simulink model "RefModel_SignalIntegrity"  (R2020a)
settings: Solver=ode1  StartTime=0.0  StopTime=10.0  FixedStep=Ts_SignalIntegrity.Ts_base  RelTol=1e-3
undefined symbols (not defined in the file or in its folder): ALGO_SET, IMU1, IMU2, IMU3, mag1, mag2, SIM_SENSOR_SET
(part 2 of 2)

== stateflow chart RefModel_SignalIntegrity/SignalIntegrityCal ==
  state FaultDetect [parallel]
    settings: executionOrder=1
    state IMU1 [parallel]
      settings: executionOrder=8
      state BaseUpdate [parallel]
        du:
        updateFlag.IMU1 = hasChanged(IN_SENSOR.IMU1.accel_x) || ...
        hasChanged(IN_SENSOR.IMU1.accel_y) || ...
        hasChanged(IN_SENSOR.IMU1.accel_z);
        settings: executionOrder=1
        state Normal
          en:
          SensorStatus.IMU1 = ENUM_SensorHealthStatus.Health;
        state Degrade
          en:
          SensorStatus.IMU1 = ENUM_SensorHealthStatus.Degrade;
        (default) -> FaultDetect.IMU1.BaseUpdate.Normal
        FaultDetect.IMU1.BaseUpdate.Degrade -> FaultDetect.IMU1.BaseUpdate.Normal : [~isMeasureAbnormal]
        FaultDetect.IMU1.BaseUpdate.Normal -> FaultDetect.IMU1.BaseUpdate.Degrade : [isMeasureAbnormal]
      state WORKING [parallel]
        settings: executionOrder=2
        state NORMAL
          en:
          sensorLostTime.IMU1 = 0;
          du:
          sensorLostTime.IMU1 = sensorLostTime.IMU1 + 1;
        state LostShort
          en:
          fprintf('\t\t\t time %.2f [sec]: IMU1 is lost shortly!\n',clock_sec);
          en,du:
          SensorStatus.IMU1 = ENUM_SensorHealthStatus.LostShort;
          sensorLostTime.IMU1 = sensorLostTime.IMU1 + 1;
        state LostLong
          en:
          fprintf('\t\t\t time %.2f [sec]: IMU1 is lost!\n',clock_sec);
          en,du:
          SensorStatus.IMU1 = ENUM_SensorHealthStatus.LostLong;
          sensorLostTime.IMU1 = sensorLostTime.IMU1 + 1;
        (default) -> FaultDetect.IMU1.WORKING.NORMAL
        (junction 288) -> FaultDetect.IMU1.WORKING.NORMAL : [updateFlag.IMU1]
            | {sensorLostTime.IMU1 = 0;}
        FaultDetect.IMU1.WORKING.NORMAL -> (junction 289) [order 1]
        FaultDetect.IMU1.WORKING.NORMAL -> FaultDetect.IMU1.WORKING.LostShort [order 2] : [sensorLostTime.IMU1 > SENSOR_INTEGRITY_PARAM.IMU.threshold_lostTime]
        (junction 289) -> (junction 288)
        (junction 290) -> (junction 288) : [updateFlag.IMU1]
            | {fprintf('\t\t\t time %.2f [sec]: IMU1 is normal!\n',clock_sec);
            | }
        FaultDetect.IMU1.WORKING.LostShort -> (junction 290) [order 1]
        FaultDetect.IMU1.WORKING.LostLong -> (junction 290)
        FaultDetect.IMU1.WORKING.LostShort -> FaultDetect.IMU1.WORKING.LostLong [order 2] : [sensorLostTime.IMU1 > 2*SENSOR_INTEGRITY_PARAM.IMU.threshold_lostTime]
    state IMU2 [parallel]
      settings: executionOrder=9
      state WORKING [parallel]
        settings: executionOrder=2
        state NORMAL
          en:
          sensorLostTime.IMU2 = 0;
          du:
          sensorLostTime.IMU2 = sensorLostTime.IMU2 + 1;
        state LostShort
          en:
          en,du:
          SensorStatus.IMU2 = ENUM_SensorHealthStatus.LostShort;
          sensorLostTime.IMU2 = sensorLostTime.IMU2 + 1;
        state LostLong
          en:
          en,du:
          SensorStatus.IMU2 = ENUM_SensorHealthStatus.LostLong;
          sensorLostTime.IMU2 = sensorLostTime.IMU2 + 1;
        (default) -> FaultDetect.IMU2.WORKING.NORMAL
        (junction 308) -> FaultDetect.IMU2.WORKING.NORMAL : [updateFlag.IMU2]
            | {sensorLostTime.IMU2 = 0;}
        FaultDetect.IMU2.WORKING.NORMAL -> (junction 309) [order 1]
        FaultDetect.IMU2.WORKING.NORMAL -> FaultDetect.IMU2.WORKING.LostShort [order 2] : [sensorLostTime.IMU2 > SENSOR_INTEGRITY_PARAM.IMU.threshold_lostTime]
        (junction 309) -> (junction 308)
        (junction 310) -> (junction 308)
        FaultDetect.IMU2.WORKING.LostShort -> (junction 310) [order 1]
        FaultDetect.IMU2.WORKING.LostLong -> (junction 310)
        FaultDetect.IMU2.WORKING.LostShort -> FaultDetect.IMU2.WORKING.LostLong [order 2] : [sensorLostTime.IMU2 > 2*SENSOR_INTEGRITY_PARAM.IMU.threshold_lostTime]
      state BaseUpdate [parallel]
        du:
        updateFlag.IMU2 = hasChanged(IN_SENSOR.IMU2.accel_x) || ...
        hasChanged(IN_SENSOR.IMU2.accel_y) || ...
        hasChanged(IN_SENSOR.IMU2.accel_z);
        if isMeasureAbnormal
        SensorStatus.IMU2 = ENUM_SensorHealthStatus.Degrade;
        else
        SensorStatus.IMU2 = ENUM_SensorHealthStatus.Health;
        end
        settings: executionOrder=1
    state IMU3 [parallel]
      settings: executionOrder=10
      state WORKING [parallel]
        settings: executionOrder=2
        state NORMAL
          en:
          sensorLostTime.IMU3 = 0;
          du:
          sensorLostTime.IMU3 = sensorLostTime.IMU3 + 1;
        state LostShort
          en:
          en,du:
          SensorStatus.IMU3 = ENUM_SensorHealthStatus.LostShort;
          sensorLostTime.IMU3 = sensorLostTime.IMU3 + 1;
        state LostLong
          en:
          en,du:
          SensorStatus.IMU3 = ENUM_SensorHealthStatus.LostLong;
          sensorLostTime.IMU3 = sensorLostTime.IMU3 + 1;
        (default) -> FaultDetect.IMU3.WORKING.NORMAL
        (junction 328) -> FaultDetect.IMU3.WORKING.NORMAL : [updateFlag.IMU3]
            | {sensorLostTime.IMU3 = 0;}
        FaultDetect.IMU3.WORKING.NORMAL -> (junction 329) [order 1]
        FaultDetect.IMU3.WORKING.NORMAL -> FaultDetect.IMU3.WORKING.LostShort [order 2] : [sensorLostTime.IMU3 > SENSOR_INTEGRITY_PARAM.IMU.threshold_lostTime]
        (junction 329) -> (junction 328)
        (junction 330) -> (junction 328)
        FaultDetect.IMU3.WORKING.LostShort -> (junction 330) [order 1]
        FaultDetect.IMU3.WORKING.LostLong -> (junction 330)
        FaultDetect.IMU3.WORKING.LostShort -> FaultDetect.IMU3.WORKING.LostLong [order 2] : [sensorLostTime.IMU3 > 2*SENSOR_INTEGRITY_PARAM.IMU.threshold_lostTime]
      state BaseUpdate [parallel]
        du:
        updateFlag.IMU3 = hasChanged(IN_SENSOR.IMU3.accel_x) || ...
        hasChanged(IN_SENSOR.IMU3.accel_y) || ...
        hasChanged(IN_SENSOR.IMU3.accel_z);
        if isMeasureAbnormal
        SensorStatus.IMU3 = ENUM_SensorHealthStatus.Degrade;
        else
        SensorStatus.IMU3 = ENUM_SensorHealthStatus.Health;
        end
        settings: executionOrder=1
    state Mag1 [parallel]
      settings: executionOrder=1
      state BaseUpdate [parallel]
        du:
        updateFlag.mag1 = hasChanged(IN_SENSOR.mag1.mag_x) || ...
        hasChanged(IN_SENSOR.mag1.mag_y) || ...
        hasChanged(IN_SENSOR.mag1.mag_z);
        settings: executionOrder=1
        state Normal
          en:
          SensorStatus.mag1 = ENUM_SensorHealthStatus.Health;
        state Degrade
          en:
          SensorStatus.mag1 = ENUM_SensorHealthStatus.Degrade;
        (default) -> FaultDetect.Mag1.BaseUpdate.Normal
        FaultDetect.Mag1.BaseUpdate.Degrade -> FaultDetect.Mag1.BaseUpdate.Normal : [~isMeasureAbnormal]
        FaultDetect.Mag1.BaseUpdate.Normal -> FaultDetect.Mag1.BaseUpdate.Degrade : [isMeasureAbnormal]
      state WORKING [parallel]
        settings: executionOrder=2
        state NORMAL
          en:
          sensorLostTime.mag1 = 0;
          SensorStatus.mag1 = ENUM_SensorHealthStatus.Health;
          du:
          sensorLostTime.mag1 = sensorLostTime.mag1 + 1;
        state LostShort
          en:
          fprintf('\t\t\t time %.2f [sec]: Mag1 is lost shortly!\n',clock_sec);
          en,du:
          SensorStatus.mag1 = ENUM_SensorHealthStatus.LostShort;
          sensorLostTime.mag1 = sensorLostTime.mag1 + 1;
        state LostLong
          en:
          fprintf('\t\t\t time %.2f [sec]: Mag1 is lost!\n',clock_sec);
          en,du:
          SensorStatus.mag1 = ENUM_SensorHealthStatus.LostLong;
          sensorLostTime.mag1 = sensorLostTime.mag1 + 1;
        (default) -> FaultDetect.Mag1.WORKING.NORMAL
        (junction 65) -> FaultDetect.Mag1.WORKING.NORMAL : [updateFlag.mag1]
            | {sensorLostTime.mag1 = 0;}
        FaultDetect.Mag1.WORKING.NORMAL -> (junction 66) [order 1]
        FaultDetect.Mag1.WORKING.NORMAL -> FaultDetect.Mag1.WORKING.LostShort [order 2] : [sensorLostTime.mag1 > SENSOR_INTEGRITY_PARAM.Mag.threshold_lostTime]
        (junction 66) -> (junction 65)
        (junction 156) -> (junction 65) : [updateFlag.mag1]
            | {
            | fprintf('\t\t\t time %.2f [sec]: Mag1 is normal!\n',clock_sec);
            | }
        FaultDetect.Mag1.WORKING.LostShort -> (junction 156) [order 1]
        FaultDetect.Mag1.WORKING.LostLong -> (junction 156)
        FaultDetect.Mag1.WORKING.LostShort -> FaultDetect.Mag1.WORKING.LostLong [order 2] : [sensorLostTime.mag1 > 2*SENSOR_INTEGRITY_PARAM.Mag.threshold_lostTime]
    state Mag2 [parallel]
      settings: executionOrder=2
      state BaseUpdate [parallel]
        du:
        updateFlag.mag2 = hasChanged(IN_SENSOR.mag2.mag_x) || ...
        hasChanged(IN_SENSOR.mag2.mag_y) || ...
        hasChanged(IN_SENSOR.mag2.mag_z);
        settings: executionOrder=1
        state Normal
          en:
          SensorStatus.mag2 = ENUM_SensorHealthStatus.Health;
        state Degrade
          en:
          SensorStatus.mag2 = ENUM_SensorHealthStatus.Degrade;
        (default) -> FaultDetect.Mag2.BaseUpdate.Normal
        FaultDetect.Mag2.BaseUpdate.Degrade -> FaultDetect.Mag2.BaseUpdate.Normal : [~isMeasureAbnormal]
        FaultDetect.Mag2.BaseUpdate.Normal -> FaultDetect.Mag2.BaseUpdate.Degrade : [isMeasureAbnormal]
      state WORKING [parallel]
        settings: executionOrder=2
        state NORMAL
          en:
          sensorLostTime.mag2 = 0;
          SensorStatus.mag2 = ENUM_SensorHealthStatus.Health;
          du:
          sensorLostTime.mag2 = sensorLostTime.mag2 + 1;
        state LostShort
          en:
          fprintf('\t\t\t time %.2f [sec]: Mag2 is lost shortly!\n',clock_sec);
          en,du:
          SensorStatus.mag2 = ENUM_SensorHealthStatus.LostShort;
          sensorLostTime.mag2 = sensorLostTime.mag2 + 1;
        state LostLong
          en:
          fprintf('\t\t\t time %.2f [sec]: Mag2 is lost!\n',clock_sec);
          en,du:
          SensorStatus.mag2 = ENUM_SensorHealthStatus.LostLong;
          sensorLostTime.mag2 = sensorLostTime.mag2 + 1;
        (default) -> FaultDetect.Mag2.WORKING.NORMAL
        (junction 168) -> FaultDetect.Mag2.WORKING.NORMAL : [updateFlag.mag2]
            | {sensorLostTime.mag2 = 0;}
        FaultDetect.Mag2.WORKING.NORMAL -> (junction 169) [order 1]
        FaultDetect.Mag2.WORKING.NORMAL -> FaultDetect.Mag2.WORKING.LostShort [order 2] : [sensorLostTime.mag2 > SENSOR_INTEGRITY_PARAM.Mag.threshold_lostTime]
        (junction 169) -> (junction 168)
        (junction 170) -> (junction 168) : [updateFlag.mag2]
            | {
            | fprintf('\t\t\t time %.2f [sec]: Mag2 is normal!\n',clock_sec);
            | }
        FaultDetect.Mag2.WORKING.LostShort -> (junction 170) [order 1]
        FaultDetect.Mag2.WORKING.LostLong -> (junction 170)
        FaultDetect.Mag2.WORKING.LostShort -> FaultDetect.Mag2.WORKING.LostLong [order 2] : [sensorLostTime.mag2 > 2*SENSOR_INTEGRITY_PARAM.Mag.threshold_lostTime]
    state Ublox1 [parallel]
      settings: executionOrder=3
      state WORKING [parallel]
        settings: executionOrder=2
        state NORMAL
          en:
          sensorLostTime.ublox1 = 0;
          du:
          sensorLostTime.ublox1 = sensorLostTime.ublox1 + 1;
        state LostShort
          en:
          fprintf('\t\t\t time %.2f [sec]: Ublox1 is lost shortly!\n',clock_sec);
          en,du:
          SensorStatus.ublox1 = ENUM_SensorHealthStatus.LostShort;
          sensorLostTime.ublox1 = sensorLostTime.ublox1 + 1;
        state LostLong
          en:
          fprintf('\t\t\t time %.2f [sec]: Ublox1 is lost!\n',clock_sec);
          en,du:
          SensorStatus.ublox1 = ENUM_SensorHealthStatus.LostLong;
          sensorLostTime.ublox1 = sensorLostTime.ublox1 + 1;
        (default) -> FaultDetect.Ublox1.WORKING.NORMAL
        (junction 188) -> FaultDetect.Ublox1.WORKING.NORMAL : [updateFlag.ublox1]
            | {sensorLostTime.ublox1 = 0;}
        FaultDetect.Ublox1.WORKING.NORMAL -> (junction 189) [order 1]
        FaultDetect.Ublox1.WORKING.NORMAL -> FaultDetect.Ublox1.WORKING.LostShort [order 2] : [sensorLostTime.ublox1 > SENSOR_INTEGRITY_PARAM.GPS.threshold_lostTime]
        (junction 189) -> (junction 188)
        (junction 190) -> (junction 188) : [updateFlag.ublox1]
            | {fprintf('\t\t\t time %.2f [sec]: Ublox1 is normal!\n',clock_sec);
            | }
        FaultDetect.Ublox1.WORKING.LostShort -> (junction 190) [order 1]
        FaultDetect.Ublox1.WORKING.LostLong -> (junction 190)
        FaultDetect.Ublox1.WORKING.LostShort -> FaultDetect.Ublox1.WORKING.LostLong [order 2] : [sensorLostTime.ublox1 > 2*SENSOR_INTEGRITY_PARAM.GPS.threshold_lostTime]
      state BaseUpdate [parallel]
        du:
        updateFlag.ublox1 = hasChanged(IN_SENSOR.ublox1.velN) || ...
        hasChanged(IN_SENSOR.ublox1.velE) || ...
        hasChanged(IN_SENSOR.ublox1.velD);
        if isMeasureAbnormal
        SensorStatus.ublox1 = ENUM_SensorHealthStatus.Degrade;
        else
        SensorStatus.ublox1 = ENUM_SensorHealthStatus.Health;
        end
        settings: executionOrder=1
    state BoardCard [parallel]
      settings: executionOrder=4
      state WORKING [parallel]
        settings: executionOrder=2
        state NORMAL
          en:
          sensorLostTime.um482 = 0;
          du:
          sensorLostTime.um482 = sensorLostTime.um482 + 1;
        state LostShort
          en,du:
          SensorStatus.um482 = ENUM_SensorHealthStatus.LostShort;
          sensorLostTime.um482 = sensorLostTime.um482 + 1;
        state LostLong
          en:
          fprintf('\t\t\t time %.2f [sec]: um482 is lost!\n',clock_sec);
          en,du:
          SensorStatus.um482 = ENUM_SensorHealthStatus.LostLong;
          sensorLostTime.um482 = sensorLostTime.um482 + 1;
        (default) -> FaultDetect.BoardCard.WORKING.NORMAL
        (junction 208) -> FaultDetect.BoardCard.WORKING.NORMAL : [updateFlag.um482]
            | {sensorLostTime.um482 = 0;}
        FaultDetect.BoardCard.WORKING.NORMAL -> (junction 209) [order 1]
        FaultDetect.BoardCard.WORKING.NORMAL -> FaultDetect.BoardCard.WORKING.LostShort [order 2] : [sensorLostTime.um482 > SENSOR_INTEGRITY_PARAM.um482.threshold_lostTime]
        (junction 209) -> (junction 208)
        (junction 210) -> (junction 208) : [updateFlag.um482]
            | {fprintf('\t\t\t time %.2f [sec]: um482 is normal!\n',clock_sec);
            | }
        FaultDetect.BoardCard.WORKING.LostShort -> (junction 210) [order 1]
        FaultDetect.BoardCard.WORKING.LostLong -> (junction 210)
        FaultDetect.BoardCard.WORKING.LostShort -> FaultDetect.BoardCard.WORKING.LostLong [order 2] : [sensorLostTime.um482 > 2*SENSOR_INTEGRITY_PARAM.um482.threshold_lostTime]
      state BaseUpdate [parallel]
        en,du:
        updateBESTPOS;
        updateFlag.um482 = hasChanged(IN_SENSOR.um482.velN) || ...
        hasChanged(IN_SENSOR.um482.velE) || ...
        hasChanged(IN_SENSOR.um482.velD);
        if isMeasureAbnormal
        SensorStatus.um482 = ENUM_SensorHealthStatus.Degrade;
        else
        SensorStatus.um482 = ENUM_SensorHealthStatus.Health;
        end
        settings: executionOrder=1
    state Baro1 [parallel]
      settings: executionOrder=5
      state WORKING [parallel]
        settings: executionOrder=2
        state NORMAL
          en:
          sensorLostTime.baro1 = 0;
          du:
          sensorLostTime.baro1 = sensorLostTime.baro1 + 1;
        state LostShort
          en:
          fprintf('\t\t\t time %.2f [sec]: Baro1 is lost shortly!\n',clock_sec);
          en,du:
          SensorStatus.baro1 = ENUM_SensorHealthStatus.LostShort;
          sensorLostTime.baro1 = sensorLostTime.baro1 + 1;
        state LostLong
          en:
          fprintf('\t\t\t time %.2f [sec]: Baro1 is lost!\n',clock_sec);
          en,du:
          SensorStatus.baro1 = ENUM_SensorHealthStatus.LostLong;
          sensorLostTime.baro1 = sensorLostTime.baro1 + 1;
        (default) -> FaultDetect.Baro1.WORKING.NORMAL
        (junction 228) -> FaultDetect.Baro1.WORKING.NORMAL : [updateFlag.baro1]
            | {sensorLostTime.baro1 = 0;}
        FaultDetect.Baro1.WORKING.NORMAL -> (junction 229) [order 1]
        FaultDetect.Baro1.WORKING.NORMAL -> FaultDetect.Baro1.WORKING.LostShort [order 2] : [sensorLostTime.baro1 > SENSOR_INTEGRITY_PARAM.Baro.threshold_lostTime]
        (junction 229) -> (junction 228)
        (junction 230) -> (junction 228) : [updateFlag.baro1]
            | {fprintf('\t\t\t time %.2f [sec]: Baro1 is normal!\n',clock_sec);
            | }
        FaultDetect.Baro1.WORKING.LostShort -> (junction 230) [order 1]
        FaultDetect.Baro1.WORKING.LostLong -> (junction 230)
        FaultDetect.Baro1.WORKING.LostShort -> FaultDetect.Baro1.WORKING.LostLong [order 2] : [sensorLostTime.baro1 > 2*SENSOR_INTEGRITY_PARAM.Baro.threshold_lostTime]
      state BaseUpdate [parallel]
        du:
        updateFlag.baro1 = hasChanged(IN_SENSOR.baro1.alt_baro);
        if isMeasureAbnormal
        SensorStatus.baro1 = ENUM_SensorHealthStatus.Degrade;
        else
        SensorStatus.baro1 = ENUM_SensorHealthStatus.Health;
        end
        settings: executionOrder=1
    state Radar1 [parallel]
      settings: executionOrder=6
      state WORKING [parallel]
        settings: executionOrder=2
        state NORMAL
          en:
          sensorLostTime.radar1 = 0;
          du:
          sensorLostTime.radar1 = sensorLostTime.radar1 + 1;
        state LostShort
          en:
          fprintf('\t\t\t time %.2f [sec]: Radar1 is lost shortly!\n',clock_sec);
          en,du:
          SensorStatus.radar1 = ENUM_SensorHealthStatus.LostShort;
          sensorLostTime.radar1 = sensorLostTime.radar1 + 1;
        state LostLong
          en:
          fprintf('\t\t\t time %.2f [sec]: Radar1 is lost!\n',clock_sec);
          en,du:
          SensorStatus.radar1 = ENUM_SensorHealthStatus.LostLong;
          sensorLostTime.radar1 = sensorLostTime.radar1 + 1;
        (default) -> FaultDetect.Radar1.WORKING.NORMAL
        (junction 248) -> FaultDetect.Radar1.WORKING.NORMAL : [updateFlag.radar1]
            | {sensorLostTime.radar1 = 0;}
        FaultDetect.Radar1.WORKING.NORMAL -> (junction 249) [order 1]
        FaultDetect.Radar1.WORKING.NORMAL -> FaultDetect.Radar1.WORKING.LostShort [order 2] : [sensorLostTime.radar1 > SENSOR_INTEGRITY_PARAM.Radar.threshold_lostTime]
        (junction 249) -> (junction 248)
        (junction 250) -> (junction 248) : [updateFlag.radar1]
            | {fprintf('\t\t\t time %.2f [sec]: Radar1 is normal!\n',clock_sec);
            | }
        FaultDetect.Radar1.WORKING.LostShort -> (junction 250) [order 1]
        FaultDetect.Radar1.WORKING.LostLong -> (junction 250)
        FaultDetect.Radar1.WORKING.LostShort -> FaultDetect.Radar1.WORKING.LostLong [order 2] : [sensorLostTime.radar1 > 2*SENSOR_INTEGRITY_PARAM.Radar.threshold_lostTime]
      state BaseUpdate [parallel]
        du:
        updateFlag.radar1 = hasChanged(IN_SENSOR.radar1.Range);
        if isMeasureAbnormal
        SensorStatus.radar1 = ENUM_SensorHealthStatus.Degrade;
        else
        SensorStatus.radar1 = ENUM_SensorHealthStatus.Health;
        end
        settings: executionOrder=1
    state Airspeed1 [parallel]
      settings: executionOrder=7
      state WORKING [parallel]
        settings: executionOrder=2
        state NORMAL
          en:
          sensorLostTime.airspeed1 = 0;
          du:
          sensorLostTime.airspeed1 = sensorLostTime.airspeed1 + 1;
        state LostShort
          en:
          fprintf('\t\t\t time %.2f [sec]: Airspeed is lost shortly!\n',clock_sec);
          en,du:
          SensorStatus.airspeed1 = ENUM_SensorHealthStatus.LostShort;
          sensorLostTime.airspeed1 = sensorLostTime.airspeed1 + 1;
        state LostLong
          en:
          fprintf('\t\t\t time %.2f [sec]: Airspeed1 is lost!\n',clock_sec);
          en,du:
          SensorStatus.airspeed1 = ENUM_SensorHealthStatus.LostLong;
          sensorLostTime.airspeed1 = sensorLostTime.airspeed1 + 1;
        (default) -> FaultDetect.Airspeed1.WORKING.NORMAL
        (junction 268) -> FaultDetect.Airspeed1.WORKING.NORMAL : [updateFlag.airspeed1]
            | {sensorLostTime.airspeed1 = 0;}
        FaultDetect.Airspeed1.WORKING.NORMAL -> (junction 269) [order 1]
        FaultDetect.Airspeed1.WORKING.NORMAL -> FaultDetect.Airspeed1.WORKING.LostShort [order 2] : [sensorLostTime.airspeed1 > SENSOR_INTEGRITY_PARAM.Airspeed.threshold_lostTime]
        (junction 269) -> (junction 268)
        (junction 270) -> (junction 268) : [updateFlag.airspeed1]
            | {fprintf('\t\t\t time %.2f [sec]: Airspeed1 is normal!\n',clock_sec);
            | }
        FaultDetect.Airspeed1.WORKING.LostShort -> (junction 270) [order 1]
        FaultDetect.Airspeed1.WORKING.LostLong -> (junction 270)
        FaultDetect.Airspeed1.WORKING.LostShort -> FaultDetect.Airspeed1.WORKING.LostLong [order 2] : [sensorLostTime.airspeed1 > 2*SENSOR_INTEGRITY_PARAM.Airspeed.threshold_lostTime]
      state BaseUpdate [parallel]
        du:
        updateFlag.airspeed1 = hasChanged(IN_SENSOR.airspeed1.airspeed);
        if isMeasureAbnormal
        SensorStatus.airspeed1 = ENUM_SensorHealthStatus.Degrade;
        else
        SensorStatus.airspeed1 = ENUM_SensorHealthStatus.Health;
        end
        settings: executionOrder=1
  state OUTPUT [parallel]
    du:
    % 信号更新
    SensorIntegrityInfo.SensorUpdateFlag = updateFlag;
    % 传感器选择
    SensorIntegrityInfo.SensorSelect = selectSensorByHealth;
    % 信号丢失信息
    SensorIntegrityInfo.sensorLostTime = sensorLostTime;
    % 信号丢失信息
    SensorIntegrityInfo.SensorStatus = SensorStatus;
    % 信号丢失信息
    SensorIntegrityInfo.SystemHealthStatus = calSystemHealthStatus;
    % ECAS
    updateECASInfo;
    settings: executionOrder=2
  data: flag function_output; flag function_output; flag function_output; flag function_output; flag function_output; flag function_output; flag function_output; flag function_output; flag function_output; flag function_output; SystemHealthStatus_out function_output; out function_output; IN_SENSOR input Bus: BUS_SENSOR size=1; SensorSelect input Bus: BUS_NAVI_SensorSignalIntegrity_SensorSelect size=1; SensorIntegrityInfo output Bus: BUS_NAVI_SensorSignalIntegrity size=1; updateFlag local Bus: BUS_NAVI_SensorSignalIntegrity_SensorUpdateFlag size=1; sensorLostTime local Bus: BUS_NAVI_SensorSignalIntegrity_sensorLostTime size=1; SENSOR_INTEGRITY_PARAM parameter Bus: BUS_SENSOR_INTEGRITY_PARAM size=1; SensorStatus local Bus: BUS_NAVI_SensorSignalIntegrity_Status size=1; clock_sec input; Ts input; ECASInfo output Bus: BUS_ECAS_SingalIntegrity size=1
  function flag = isMeasureAbnormal:
    | function flag = isMeasureAbnormal
    | flag = false;
  function flag = isMeasureAbnormal:
    | function flag = isMeasureAbnormal
    | flag = false;
  function flag = isMeasureAbnormal:
    | function flag = isMeasureAbnormal
    | flag = false;
  function flag = isMeasureAbnormal:
    | function flag = isMeasureAbnormal
    | persistent normMag_pre maxMag_pre minMag_pre errIdx
    | normMag = double(norm([IN_SENSOR.mag1.mag_x,IN_SENSOR.mag1.mag_y,IN_SENSOR.mag1.mag_z]));
    | if isempty(normMag_pre)
    |     normMag_pre = normMag;
    |     maxMag_pre = normMag;
    |     minMag_pre = normMag;
    |     errIdx = 0;
    | end
    | if normMag < minMag_pre % 更新最小值
    |     minMag_pre = normMag;
    | end
    | if normMag > maxMag_pre % 更新最大值
    |     maxMag_pre = normMag;
    | end
    | flag = false;
    | if normMag < SENSOR_INTEGRITY_PARAM.Mag.threshold_minNormMag_uT || ...
    |         normMag > SENSOR_INTEGRITY_PARAM.Mag.threshold_maxNormMag_uT || ...
    |            normMag - normMag_pre > SENSOR_INTEGRITY_PARAM.Mag.threshold_gapBetweenMaxMin_uT
    |     errIdx = errIdx + Ts;
    |     if errIdx > 1
    |         flag = true; 
    |     end
    | end
    | normMag_pre = normMag;
  function flag = isMeasureAbnormal:
    | function flag = isMeasureAbnormal
    | persistent normMag_pre maxMag_pre minMag_pre errIdx
    | normMag = double(norm([IN_SENSOR.mag2.mag_x,IN_SENSOR.mag2.mag_y,IN_SENSOR.mag2.mag_z]));
    | if isempty(normMag_pre)
    |     normMag_pre = normMag;
    |     maxMag_pre = normMag;
    |     minMag_pre = normMag;
    |     errIdx = 0;
    | end
    | if normMag < minMag_pre % 更新最小值
    |     minMag_pre = normMag;
    | end
    | if normMag > maxMag_pre % 更新最大值
    |     maxMag_pre = normMag;
    | end
    | flag = false;
    | if normMag < SENSOR_INTEGRITY_PARAM.Mag.threshold_minNormMag_uT || ...
    |         normMag > SENSOR_INTEGRITY_PARAM.Mag.threshold_maxNormMag_uT || ...
    |            normMag - normMag_pre > SENSOR_INTEGRITY_PARAM.Mag.threshold_gapBetweenMaxMin_uT
    |     errIdx = errIdx + Ts;
    |     if errIdx > 1
    |         flag = true; 
    |     end
    | end
    | normMag_pre = normMag;
  function flag = isMeasureAbnormal:
    | function flag = isMeasureAbnormal
    | persistent lat_pre lon_pre speed_pre errIdx
    | tempGPS = IN_SENSOR.ublox1;
    | curLat = double(tempGPS.Lat);
    | curLon = double(tempGPS.Lon);
    | curSpeed = double(norm([tempGPS.velN,tempGPS.velE,tempGPS.velD]));
    | if isempty(lat_pre)
    |     lat_pre = curLat;
    |     lon_pre = curLon;
    |     speed_pre = curSpeed;
    |     errIdx = 0;
    | end
    | 
    | flag = false;
    | if tempGPS.numSv < SENSOR_INTEGRITY_PARAM.GPS.threshold_numSv || ...
    |         tempGPS.pDop > SENSOR_INTEGRITY_PARAM.GPS.threshold_pDop || ...
    |         abs(lat_pre-curLat) > 5e-4 || ...
    |         abs(lon_pre-curLon) > 5e-4 || ...
    |         abs(speed_pre-curSpeed) > 10
    |     errIdx = errIdx + Ts;
    |     if errIdx > 5
    |         flag = true; 
    |     end
    | else
    |     errIdx = 0;
    | end
    | 
    | lat_pre = curLat;
    | lon_pre = curLon;
    | speed_pre = curSpeed;
  function flag = isMeasureAbnormal:
    | function flag = isMeasureAbnormal
    | persistent lat_pre lon_pre speed_pre errIdx
    | tempGPS = IN_SENSOR.um482;
    | curLat = double(tempGPS.Lat);
    | curLon = double(tempGPS.Lon);
    | curSpeed = double(norm([tempGPS.velN,tempGPS.velE,tempGPS.velD]));
    | if isempty(lat_pre)
    |     lat_pre = curLat;
    |     lon_pre = curLon;
    |     speed_pre = curSpeed;
    |     errIdx = 0;
    | end
    | 
    | flag = false;
    | if tempGPS.numSv < SENSOR_INTEGRITY_PARAM.um482.threshold_numSv || ...
    |         tempGPS.pDop > SENSOR_INTEGRITY_PARAM.um482.threshold_pDop || ...
    |         abs(lat_pre-curLat) > 5e-4 || ...
    |         abs(lon_pre-curLon) > 5e-4 || ...
    |         abs(speed_pre-curSpeed) > 20
    |     errIdx = errIdx + Ts;
    |     if errIdx > 5
    |         flag = true; 
    |     end
    | else
    |     errIdx = 0;
    | end
    | 
    | lat_pre = curLat;
    | lon_pre = curLon;
    | speed_pre = curSpeed;
  function updateBESTPOS:
    | function updateBESTPOS
  function flag = isMeasureAbnormal:
    | function flag = isMeasureAbnormal
    | persistent preHeight
    | if isempty(preHeight)
    |     preHeight = 0; 
    | end
    | flag = false;
    | if abs(preHeight-IN_SENSOR.baro1.alt_baro) > 10
    |     flag = true; 
    | end
    | preHeight = double(IN_SENSOR.baro1.alt_baro);
  function flag = isMeasureAbnormal:
    | function flag = isMeasureAbnormal
    | persistent preVal
    | if isempty(preVal)
    |     preVal = IN_SENSOR.radar1.Range;
    | end
    | flag = false;
    | if abs(preVal-IN_SENSOR.radar1.Range)>10
    |     flag = true;
    | end
    | preVal = IN_SENSOR.radar1.Range;
  function flag = isMeasureAbnormal:
    | function flag = isMeasureAbnormal
    | flag = false;
  function SystemHealthStatus_out = calSystemHealthStatus:
    | function SystemHealthStatus_out = calSystemHealthStatus
    | SystemHealthStatus_out = ENUM_SystemHealthStatus.SystemHealth;
    | if SensorIntegrityInfo.SensorStatus.IMU1 == ENUM_SensorHealthStatus.Health && ...
    |         (SensorIntegrityInfo.SensorStatus.ublox1 == ENUM_SensorHealthStatus.Health)
    |     %         SensorIntegrityInfo.SensorStatus.mag2 == ENUM_SensorHealthStatus.Health && ...
    |     %         SensorIntegrityInfo.SensorStatus.baro1 == ENUM_SensorHealthStatus.Health
    |     SystemHealthStatus_out = ENUM_SystemHealthStatus.SystemHealth;
    | elseif SensorIntegrityInfo.SensorStatus.IMU1 == ENUM_SensorHealthStatus.Health && ...
    |         (SensorIntegrityInfo.SensorStatus.ublox1 ~= ENUM_SensorHealthStatus.Health && ...
    |          SensorIntegrityInfo.SensorStatus.um482 == ENUM_SensorHealthStatus.Health)
    |     SystemHealthStatus_out = ENUM_SystemHealthStatus.DontTakeOff;
    | else
    |     SystemHealthStatus_out = ENUM_SystemHealthStatus.CanNotFly;
    | end
  function out = selectSensorByHealth:
    | function out = selectSensorByHealth
    | out = SensorSelect;
    | %% 磁力计信号优选
    | if SensorStatus.mag2 == ENUM_SensorHealthStatus.Health % 磁力计2健康
    |     out.Mag = single(2);
    | elseif  SensorStatus.mag1 == ENUM_SensorHealthStatus.Health
    |     out.Mag = single(1);
    | else
    |     out.Mag = single(-1);
    | end
  function updateECASInfo:
    | function updateECASInfo
    | % 磁力计
    | if SensorStatus.mag1 == ENUM_SensorHealthStatus.Degrade || ...
    |         SensorStatus.mag2 == ENUM_SensorHealthStatus.Degrade
    |     ECASInfo.anyDegrade_mag = int8(1);
    | end
    | % 
    | mag1Val = [IN_SENSOR.mag1.mag_x,IN_SENSOR.mag1.mag_y,IN_SENSOR.mag1.mag_z];
    | mag2Val = [IN_SENSOR.mag2.mag_x,IN_SENSOR.mag2.mag_y,IN_SENSOR.mag2.mag_z];
    | if norm(mag1Val-mag2Val) > 0.15*min(norm(mag1Val),norm(mag2Val))
    |     ECASInfo.precisionMismatch_mag = int8(1);
    | end
  function getSensorSignalBySelect:
    | function getSensorSignalBySelect
    | % IMU更新
    | if SensorIntegrityInfo.SensorSelect.IMU == 1
    |     imuUpdateFlag = SensorIntegrityInfo.SensorUpdateFlag.IMU1;
    |     accel = IMU1_accel;
    |     gyro = IMU1_gyro;
    | elseif SensorIntegrityInfo.SensorSelect.IMU == 2
    |     imuUpdateFlag = SensorIntegrityInfo.SensorUpdateFlag.IMU2;
    |     accel = IMU2_accel;
    |     gyro = IMU2_gyro;
    | elseif SensorIntegrityInfo.SensorSelect.IMU == 3
    |     imuUpdateFlag = SensorIntegrityInfo.SensorUpdateFlag.IMU3;
    |     accel = IMU3_accel;
    |     gyro = IMU3_gyro;
    | elseif SensorIntegrityInfo.SensorSelect.IMU == 0
    |     imuUpdateFlag = SensorIntegrityInfo.SensorUpdateFlag.IMU1 & SensorIntegrityInfo.SensorUpdateFlag.IMU2 & SensorIntegrityInfo.SensorUpdateFlag.IMU3;
    |     accel = (IMU1_accel+IMU2_accel+IMU3_accel)/3;
    |     gyro = (IMU1_gyro+IMU2_gyro+IMU3_gyro)/3;
    | else
    |     imuUpdateFlag = true;
    |     accelTemp = single([0,0,0]);
    |     gyroTemp = single([0,0,0]);
    |     error('IMU config error')
    | end
    | % Mag更新
    | if SensorIntegrityInfo.SensorSelect.Mag == 1
    |     magUpdateFlag = SensorIntegrityInfo.SensorUpdateFlag.mag1;
    |     mag = mag1;
    | elseif SensorIntegrityInfo.SensorSelect.Mag == 2
    |     magUpdateFlag = SensorIntegrityInfo.SensorUpdateFlag.mag2;
    |     mag = mag2;
    | elseif SensorIntegrityInfo.SensorSelect.Mag == 0
    |     magUpdateFlag = SensorIntegrityInfo.SensorUpdateFlag.mag1 & SensorIntegrityInfo.SensorUpdateFlag.mag2;
    |     mag = (mag1+mag2)/2;
    | else % 随便预置一个地磁矢量
    |     magUpdateFlag = true;
    |     mag = [1,0,0];
    | end
    | % GPS更新
    | lla = ublox1_lla;
    | gpsvel = ublox1_gpsvel;
    | gpsUpdateFlag = SensorIntegrityInfo.SensorUpdateFlag.ublox1;
    | % 气压高度计更新
    | alt = baro1_alt;
    | baroUpdateFlag = SensorIntegrityInfo.SensorUpdateFlag.baro1;
    | % 雷达高度计更新
    | range = radar1_range;
    | radarUpdateFlag = SensorIntegrityInfo.SensorUpdateFlag.radar1;

== stateflow chart RefModel_SignalIntegrity/updateFlag ==
  state BaseUpdateTick [parallel] [commented out]
    en:
    baseTick = 0;
    du:
    baseTick = baseTick + 1;
  state FaultDetect [parallel] [commented out]
    state IMU1 [parallel] [commented out]
      state WORKING [parallel] [commented out]
        state NORMAL [commented out]
          en:
          sensorLostTime.IMU1 = 0;
          du:
          sensorLostTime.IMU1 = sensorLostTime.IMU1 + 1;
        state LostShort [commented out]
          en:
          du:
          SensorStatus.IMU1 = ENUM_SensorHealthStatus.LostShort;
          sensorLostTime.IMU1 = sensorLostTime.IMU1 + 1;
        state LostLong [commented out]
          en:
          du:
          SensorStatus.IMU1 = ENUM_SensorHealthStatus.LostLong;
          sensorLostTime.IMU1 = sensorLostTime.IMU1 + 1;
        (default) -> FaultDetect.IMU1.WORKING.NORMAL [commented out]
        (junction 288) -> FaultDetect.IMU1.WORKING.NORMAL [commented out] : [updateFlag.IMU1]
            | {sensorLostTime.IMU1 = 0;}
        FaultDetect.IMU1.WORKING.NORMAL -> (junction 289) [commented out]
        FaultDetect.IMU1.WORKING.NORMAL -> FaultDetect.IMU1.WORKING.LostShort [commented out] : [sensorLostTime.IMU1 > SENSOR_INTEGRITY_PARAM.IMU.threshold_lostTime]
        (junction 289) -> (junction 288) [commented out]
        (junction 290) -> (junction 288) [commented out]
        FaultDetect.IMU1.WORKING.LostShort -> (junction 290) [commented out]
        FaultDetect.IMU1.WORKING.LostLong -> (junction 290) [commented out]
        FaultDetect.IMU1.WORKING.LostShort -> FaultDetect.IMU1.WORKING.LostLong [commented out] : [sensorLostTime.IMU1 > 2*SENSOR_INTEGRITY_PARAM.IMU.threshold_lostTime]
      state BaseUpdate [parallel] [commented out]
        du:
        updateFlag.IMU1 = hasChanged(IN_SENSOR.IMU1.accel_x) || ...
        hasChanged(IN_SENSOR.IMU1.accel_y) || ...
        hasChanged(IN_SENSOR.IMU1.accel_z);
        if isMeasureAbnormal
        SensorStatus.IMU1 = ENUM_SensorHealthStatus.Degrade;
        else
        SensorStatus.IMU1 = ENUM_SensorHealthStatus.Health;
        end
    state IMU2 [parallel] [commented out]
      state WORKING [parallel] [commented out]
        state NORMAL [commented out]
          en:
          sensorLostTime.IMU2 = 0;
          du:
          sensorLostTime.IMU2 = sensorLostTime.IMU2 + 1;
        state LostShort [commented out]
          en:
          du:
          SensorStatus.IMU2 = ENUM_SensorHealthStatus.LostShort;
          sensorLostTime.IMU2 = sensorLostTime.IMU2 + 1;
        state LostLong [commented out]
          en:
          du:
          SensorStatus.IMU2 = ENUM_SensorHealthStatus.LostLong;
          sensorLostTime.IMU2 = sensorLostTime.IMU2 + 1;
        (default) -> FaultDetect.IMU2.WORKING.NORMAL [commented out]
        (junction 308) -> FaultDetect.IMU2.WORKING.NORMAL [commented out] : [updateFlag.IMU2]
            | {sensorLostTime.IMU2 = 0;}
        FaultDetect.IMU2.WORKING.NORMAL -> (junction 309) [commented out]
        FaultDetect.IMU2.WORKING.NORMAL -> FaultDetect.IMU2.WORKING.LostShort [commented out] : [sensorLostTime.IMU2 > SENSOR_INTEGRITY_PARAM.IMU.threshold_lostTime]
        (junction 309) -> (junction 308) [commented out]
        (junction 310) -> (junction 308) [commented out]
        FaultDetect.IMU2.WORKING.LostShort -> (junction 310) [commented out]
        FaultDetect.IMU2.WORKING.LostLong -> (junction 310) [commented out]
        FaultDetect.IMU2.WORKING.LostShort -> FaultDetect.IMU2.WORKING.LostLong [commented out] : [sensorLostTime.IMU2 > 2*SENSOR_INTEGRITY_PARAM.IMU.threshold_lostTime]
      state BaseUpdate [parallel] [commented out]
        du:
        updateFlag.IMU2 = hasChanged(IN_SENSOR.IMU2.accel_x) || ...
        hasChanged(IN_SENSOR.IMU2.accel_y) || ...
        hasChanged(IN_SENSOR.IMU2.accel_z);
        if isMeasureAbnormal
        SensorStatus.IMU2 = ENUM_SensorHealthStatus.Degrade;
        else
        SensorStatus.IMU2 = ENUM_SensorHealthStatus.Health;
        end
    state IMU3 [parallel] [commented out]
      state WORKING [parallel] [commented out]
        state NORMAL [commented out]
          en:
          sensorLostTime.IMU3 = 0;
          du:
          sensorLostTime.IMU3 = sensorLostTime.IMU3 + 1;
        state LostShort [commented out]
          en:
          du:
          SensorStatus.IMU3 = ENUM_SensorHealthStatus.LostShort;
          sensorLostTime.IMU3 = sensorLostTime.IMU3 + 1;
        state LostLong [commented out]
          en:
          du:
          SensorStatus.IMU3 = ENUM_SensorHealthStatus.LostLong;
          sensorLostTime.IMU3 = sensorLostTime.IMU3 + 1;
        (default) -> FaultDetect.IMU3.WORKING.NORMAL [commented out]
        (junction 328) -> FaultDetect.IMU3.WORKING.NORMAL [commented out] : [updateFlag.IMU3]
            | {sensorLostTime.IMU3 = 0;}
        FaultDetect.IMU3.WORKING.NORMAL -> (junction 329) [commented out]
        FaultDetect.IMU3.WORKING.NORMAL -> FaultDetect.IMU3.WORKING.LostShort [commented out] : [sensorLostTime.IMU3 > SENSOR_INTEGRITY_PARAM.IMU.threshold_lostTime]
        (junction 329) -> (junction 328) [commented out]
        (junction 330) -> (junction 328) [commented out]
        FaultDetect.IMU3.WORKING.LostShort -> (junction 330) [commented out]
        FaultDetect.IMU3.WORKING.LostLong -> (junction 330) [commented out]
        FaultDetect.IMU3.WORKING.LostShort -> FaultDetect.IMU3.WORKING.LostLong [commented out] : [sensorLostTime.IMU3 > 2*SENSOR_INTEGRITY_PARAM.IMU.threshold_lostTime]
      state BaseUpdate [parallel] [commented out]
        du:
        updateFlag.IMU3 = hasChanged(IN_SENSOR.IMU3.accel_x) || ...
        hasChanged(IN_SENSOR.IMU3.accel_y) || ...
        hasChanged(IN_SENSOR.IMU3.accel_z);
        if isMeasureAbnormal
        SensorStatus.IMU3 = ENUM_SensorHealthStatus.Degrade;
        else
        SensorStatus.IMU3 = ENUM_SensorHealthStatus.Health;
        end
    state Mag1 [parallel] [commented out]
      state WORKING [parallel] [commented out]
        state NORMAL [commented out]
          en:
          sensorLostTime.mag1 = 0;
          du:
          sensorLostTime.mag1 = sensorLostTime.mag1 + 1;
        state LostShort [commented out]
          du:
          SensorStatus.mag1 = ENUM_SensorHealthStatus.LostShort;
          sensorLostTime.mag1 = sensorLostTime.mag1 + 1;
        state LostLong [commented out]
          du:
          SensorStatus.mag1 = ENUM_SensorHealthStatus.LostLong;
          sensorLostTime.mag1 = sensorLostTime.mag1 + 1;
        (default) -> FaultDetect.Mag1.WORKING.NORMAL [commented out]
        (junction 65) -> FaultDetect.Mag1.WORKING.NORMAL [commented out] : [updateFlag.mag1]
            | {sensorLostTime.mag1 = 0;}
        FaultDetect.Mag1.WORKING.NORMAL -> (junction 66) [commented out]
        FaultDetect.Mag1.WORKING.NORMAL -> FaultDetect.Mag1.WORKING.LostShort [commented out] : [sensorLostTime.mag1 > SENSOR_INTEGRITY_PARAM.Mag.threshold_lostTime]
        (junction 66) -> (junction 65) [commented out]
        (junction 156) -> (junction 65) [commented out]
        FaultDetect.Mag1.WORKING.LostShort -> (junction 156) [commented out]
        FaultDetect.Mag1.WORKING.LostLong -> (junction 156) [commented out]
        FaultDetect.Mag1.WORKING.LostShort -> FaultDetect.Mag1.WORKING.LostLong [commented out] : [sensorLostTime.mag1 > 2*SENSOR_INTEGRITY_PARAM.Mag.threshold_lostTime]
      state BaseUpdate [parallel] [commented out]
        du:
        updateFlag.mag1 = hasChanged(IN_SENSOR.mag1.mag_x) || ...
        hasChanged(IN_SENSOR.mag1.mag_y) || ...
        hasChanged(IN_SENSOR.mag1.mag_z);
        if isMeasureAbnormal
        SensorStatus.mag1 = ENUM_SensorHealthStatus.Degrade;
        else
        SensorStatus.mag1 = ENUM_SensorHealthStatus.Health;
        end
    state Mag2 [parallel] [commented out]
      state WORKING [parallel] [commented out]
        state NORMAL [commented out]
          en:
          sensorLostTime.mag2 = 0;
          du:
          sensorLostTime.mag2 = sensorLostTime.mag2 + 1;
        state LostShort [commented out]
          du:
          SensorStatus.mag2 = ENUM_SensorHealthStatus.LostShort;
          sensorLostTime.mag2 = sensorLostTime.mag2 + 1;
        state LostLong [commented out]
          du:
          SensorStatus.mag2 = ENUM_SensorHealthStatus.LostLong;
          sensorLostTime.mag2 = sensorLostTime.mag2 + 1;
        (default) -> FaultDetect.Mag2.WORKING.NORMAL [commented out]
        (junction 168) -> FaultDetect.Mag2.WORKING.NORMAL [commented out] : [updateFlag.mag2]
            | {sensorLostTime.mag2 = 0;}
        FaultDetect.Mag2.WORKING.NORMAL -> (junction 169) [commented out]
        FaultDetect.Mag2.WORKING.NORMAL -> FaultDetect.Mag2.WORKING.LostShort [commented out] : [sensorLostTime.mag2 > SENSOR_INTEGRITY_PARAM.Mag.threshold_lostTime]
        (junction 169) -> (junction 168) [commented out]
        (junction 170) -> (junction 168) [commented out]
        FaultDetect.Mag2.WORKING.LostShort -> (junction 170) [commented out]
        FaultDetect.Mag2.WORKING.LostLong -> (junction 170) [commented out]
        FaultDetect.Mag2.WORKING.LostShort -> FaultDetect.Mag2.WORKING.LostLong [commented out] : [sensorLostTime.mag2 > 2*SENSOR_INTEGRITY_PARAM.Mag.threshold_lostTime]
      state BaseUpdate [parallel] [commented out]
        du:
        updateFlag.mag2 = hasChanged(IN_SENSOR.mag2.mag_x) || ...
        hasChanged(IN_SENSOR.mag2.mag_y) || ...
        hasChanged(IN_SENSOR.mag2.mag_z);
        if isMeasureAbnormal
        SensorStatus.mag2 = ENUM_SensorHealthStatus.Degrade;
        else
        SensorStatus.mag2 = ENUM_SensorHealthStatus.Health;
        end
    state Ublox1 [parallel] [commented out]
      state WORKING [parallel] [commented out]
        state NORMAL [commented out]
          en:
          sensorLostTime.ublox1 = 0;
          du:
          sensorLostTime.ublox1 = sensorLostTime.ublox1 + 1;
        state LostShort [commented out]
          du:
          SensorStatus.ublox1 = ENUM_SensorHealthStatus.LostShort;
          sensorLostTime.ublox1 = sensorLostTime.ublox1 + 1;
        state LostLong [commented out]
          du:
          SensorStatus.ublox1 = ENUM_SensorHealthStatus.LostLong;
          sensorLostTime.ublox1 = sensorLostTime.ublox1 + 1;
        (default) -> FaultDetect.Ublox1.WORKING.NORMAL [commented out]
        (junction 188) -> FaultDetect.Ublox1.WORKING.NORMAL [commented out] : [updateFlag.ublox1]
            | {sensorLostTime.ublox1 = 0;}
        FaultDetect.Ublox1.WORKING.NORMAL -> (junction 189) [commented out]
        FaultDetect.Ublox1.WORKING.NORMAL -> FaultDetect.Ublox1.WORKING.LostShort [commented out] : [sensorLostTime.ublox1 > SENSOR_INTEGRITY_PARAM.GPS.threshold_lostTime]
        (junction 189) -> (junction 188) [commented out]
        (junction 190) -> (junction 188) [commented out]
        FaultDetect.Ublox1.WORKING.LostShort -> (junction 190) [commented out]
        FaultDetect.Ublox1.WORKING.LostLong -> (junction 190) [commented out]
        FaultDetect.Ublox1.WORKING.LostShort -> FaultDetect.Ublox1.WORKING.LostLong [commented out] : [sensorLostTime.ublox1 > 2*SENSOR_INTEGRITY_PARAM.GPS.threshold_lostTime]
      state BaseUpdate [parallel] [commented out]
        du:
        updateFlag.ublox1 = hasChanged(IN_SENSOR.ublox1.velN) || ...
        hasChanged(IN_SENSOR.ublox1.velE) || ...
        hasChanged(IN_SENSOR.ublox1.velD);
        if isMeasureAbnormal
        SensorStatus.ublox1 = ENUM_SensorHealthStatus.Degrade;
        else
        SensorStatus.ublox1 = ENUM_SensorHealthStatus.Health;
        end
    state BoardCard [parallel] [commented out]
      state WORKING [parallel] [commented out]
        state NORMAL [commented out]
          en:
          sensorLostTime.um482 = 0;
          du:
          sensorLostTime.um482 = sensorLostTime.um482 + 1;
        state LostShort [commented out]
          du:
          SensorStatus.um482 = ENUM_SensorHealthStatus.LostShort;
          sensorLostTime.um482 = sensorLostTime.um482 + 1;
        state LostLong [commented out]
          du:
          SensorStatus.um482 = ENUM_SensorHealthStatus.LostLong;
          sensorLostTime.um482 = sensorLostTime.um482 + 1;
        (default) -> FaultDetect.BoardCard.WORKING.NORMAL [commented out]
        (junction 208) -> FaultDetect.BoardCard.WORKING.NORMAL [commented out] : [updateFlag.um482]
            | {sensorLostTime.um482 = 0;}
        FaultDetect.BoardCard.WORKING.NORMAL -> (junction 209) [commented out]
        FaultDetect.BoardCard.WORKING.NORMAL -> FaultDetect.BoardCard.WORKING.LostShort [commented out] : [sensorLostTime.um482 > SENSOR_INTEGRITY_PARAM.GPS.threshold_lostTime]
        (junction 209) -> (junction 208) [commented out]
        (junction 210) -> (junction 208) [commented out]
        FaultDetect.BoardCard.WORKING.LostShort -> (junction 210) [commented out]
        FaultDetect.BoardCard.WORKING.LostLong -> (junction 210) [commented out]
        FaultDetect.BoardCard.WORKING.LostShort -> FaultDetect.BoardCard.WORKING.LostLong [commented out] : [sensorLostTime.um482 > 2*SENSOR_INTEGRITY_PARAM.GPS.threshold_lostTime]
      state BaseUpdate [parallel] [commented out]
        du:
        updateFlag.um482 = hasChanged(IN_SENSOR.um482.velN) || ...
        hasChanged(IN_SENSOR.um482.velE) || ...
        hasChanged(IN_SENSOR.um482.velD);
        if isMeasureAbnormal
        SensorStatus.um482 = ENUM_SensorHealthStatus.Degrade;
        else
        SensorStatus.um482 = ENUM_SensorHealthStatus.Health;
        end
    state Baro1 [parallel] [commented out]
      state WORKING [parallel] [commented out]
        state NORMAL [commented out]
          en:
          sensorLostTime.baro1 = 0;
          du:
          sensorLostTime.baro1 = sensorLostTime.baro1 + 1;
        state LostShort [commented out]
          en:
          du:
          SensorStatus.baro1 = ENUM_SensorHealthStatus.LostShort;
          sensorLostTime.baro1 = sensorLostTime.baro1 + 1;
        state LostLong [commented out]
          en:
          du:
          SensorStatus.baro1 = ENUM_SensorHealthStatus.LostLong;
          sensorLostTime.baro1 = sensorLostTime.baro1 + 1;
        (default) -> FaultDetect.Baro1.WORKING.NORMAL [commented out]
        (junction 228) -> FaultDetect.Baro1.WORKING.NORMAL [commented out] : [updateFlag.baro1]
            | {sensorLostTime.baro1 = 0;}
        FaultDetect.Baro1.WORKING.NORMAL -> (junction 229) [commented out]
        FaultDetect.Baro1.WORKING.NORMAL -> FaultDetect.Baro1.WORKING.LostShort [commented out] : [sensorLostTime.baro1 > SENSOR_INTEGRITY_PARAM.Baro.threshold_lostTime]
        (junction 229) -> (junction 228) [commented out]
        (junction 230) -> (junction 228) [commented out]
        FaultDetect.Baro1.WORKING.LostShort -> (junction 230) [commented out]
        FaultDetect.Baro1.WORKING.LostLong -> (junction 230) [commented out]
        FaultDetect.Baro1.WORKING.LostShort -> FaultDetect.Baro1.WORKING.LostLong [commented out] : [sensorLostTime.baro1 > 2*SENSOR_INTEGRITY_PARAM.Baro.threshold_lostTime]
      state BaseUpdate [parallel] [commented out]
        du:
        updateFlag.baro1 = hasChanged(IN_SENSOR.baro1.alt_baro);
        if isMeasureAbnormal
        SensorStatus.baro1 = ENUM_SensorHealthStatus.Degrade;
        else
        SensorStatus.baro1 = ENUM_SensorHealthStatus.Health;
        end
    state Radar1 [parallel] [commented out]
      state WORKING [parallel] [commented out]
        state NORMAL [commented out]
          en:
          sensorLostTime.radar1 = 0;
          du:
          sensorLostTime.radar1 = sensorLostTime.radar1 + 1;
        state LostShort [commented out]
          en:
          du:
          SensorStatus.radar1 = ENUM_SensorHealthStatus.LostShort;
          sensorLostTime.radar1 = sensorLostTime.radar1 + 1;
        state LostLong [commented out]
          en:
          du:
          SensorStatus.radar1 = ENUM_SensorHealthStatus.LostLong;
          sensorLostTime.radar1 = sensorLostTime.radar1 + 1;
        (default) -> FaultDetect.Radar1.WORKING.NORMAL [commented out]
        (junction 248) -> FaultDetect.Radar1.WORKING.NORMAL [commented out] : [updateFlag.radar1]
            | {sensorLostTime.radar1 = 0;}
        FaultDetect.Radar1.WORKING.NORMAL -> (junction 249) [commented out]
        FaultDetect.Radar1.WORKING.NORMAL -> FaultDetect.Radar1.WORKING.LostShort [commented out] : [sensorLostTime.radar1 > SENSOR_INTEGRITY_PARAM.Radar.threshold_lostTime]
        (junction 249) -> (junction 248) [commented out]
        (junction 250) -> (junction 248) [commented out]
        FaultDetect.Radar1.WORKING.LostShort -> (junction 250) [commented out]
        FaultDetect.Radar1.WORKING.LostLong -> (junction 250) [commented out]
        FaultDetect.Radar1.WORKING.LostShort -> FaultDetect.Radar1.WORKING.LostLong [commented out] : [sensorLostTime.radar1 > 2*SENSOR_INTEGRITY_PARAM.Radar.threshold_lostTime]
      state BaseUpdate [parallel] [commented out]
        du:
        updateFlag.radar1 = hasChanged(IN_SENSOR.radar1.Range);
        if isMeasureAbnormal
        SensorStatus.radar1 = ENUM_SensorHealthStatus.Degrade;
        else
        SensorStatus.radar1 = ENUM_SensorHealthStatus.Health;
        end
    state Airspeed1 [parallel] [commented out]
      state WORKING [parallel] [commented out]
        state NORMAL [commented out]
          en:
          sensorLostTime.airspeed1 = 0;
          du:
          sensorLostTime.airspeed1 = sensorLostTime.airspeed1 + 1;
        state LostShort [commented out]
          en:
          du:
          SensorStatus.airspeed1 = ENUM_SensorHealthStatus.LostShort;
          sensorLostTime.airspeed1 = sensorLostTime.airspeed1 + 1;
        state LostLong [commented out]
          en:
          du:
          SensorStatus.airspeed1 = ENUM_SensorHealthStatus.LostLong;
          sensorLostTime.airspeed1 = sensorLostTime.airspeed1 + 1;
        (default) -> FaultDetect.Airspeed1.WORKING.NORMAL [commented out]
        (junction 268) -> FaultDetect.Airspeed1.WORKING.NORMAL [commented out] : [updateFlag.airspeed1]
            | {sensorLostTime.airspeed1 = 0;}
        FaultDetect.Airspeed1.WORKING.NORMAL -> (junction 269) [commented out]
        FaultDetect.Airspeed1.WORKING.NORMAL -> FaultDetect.Airspeed1.WORKING.LostShort [commented out] : [sensorLostTime.airspeed1 > SENSOR_INTEGRITY_PARAM.Airspeed.threshold_lostTime]
        (junction 269) -> (junction 268) [commented out]
        (junction 270) -> (junction 268) [commented out]
        FaultDetect.Airspeed1.WORKING.LostShort -> (junction 270) [commented out]
        FaultDetect.Airspeed1.WORKING.LostLong -> (junction 270) [commented out]
        FaultDetect.Airspeed1.WORKING.LostShort -> FaultDetect.Airspeed1.WORKING.LostLong [commented out] : [sensorLostTime.airspeed1 > 2*SENSOR_INTEGRITY_PARAM.Airspeed.threshold_lostTime]
      state BaseUpdate [parallel] [commented out]
        du:
        updateFlag.airspeed1 = hasChanged(IN_SENSOR.airspeed1.airspeed);
        if isMeasureAbnormal
        SensorStatus.airspeed1 = ENUM_SensorHealthStatus.Degrade;
        else
        SensorStatus.airspeed1 = ENUM_SensorHealthStatus.Health;
        end
  state updateDetermine [parallel]
    du:
    % 传感器更新判定
    updateFlag.mag1 = hasChanged(IN_SENSOR.mag1.mag_x) || ...
    hasChanged(IN_SENSOR.mag1.mag_y) || ...
    hasChanged(IN_SENSOR.mag1.mag_z);
    updateFlag.mag2 = hasChanged(IN_SENSOR.mag2.mag_x) || ...
    hasChanged(IN_SENSOR.mag2.mag_y) || ...
    hasChanged(IN_SENSOR.mag2.mag_z);
    updateFlag.um482 = hasChanged(IN_SENSOR.um482.velN) || ...
    hasChanged(IN_SENSOR.um482.velE) || ...
    hasChanged(IN_SENSOR.um482.velD);
    updateFlag.airspeed1 = hasChanged(IN_SENSOR.airspeed1.airspeed);
    updateFlag.radar1 = hasChanged(IN_SENSOR.radar1.Range);
    updateFlag.ublox1 = hasChanged(IN_SENSOR.ublox1.velN) || ...
    hasChanged(IN_SENSOR.ublox1.velE) || ...
    hasChanged(IN_SENSOR.ublox1.velD);
    updateFlag.IMU1 = hasChanged(IN_SENSOR.IMU1.accel_x) || ...
    hasChanged(IN_SENSOR.IMU1.accel_y) || ...
    hasChanged(IN_SENSOR.IMU1.accel_z);
    updateFlag.IMU2 = hasChanged(IN_SENSOR.IMU2.accel_x) || ...
    hasChanged(IN_SENSOR.IMU2.accel_y) || ...
    hasChanged(IN_SENSOR.IMU2.accel_z);
    updateFlag.IMU3 = hasChanged(IN_SENSOR.IMU3.accel_x) || ...
    hasChanged(IN_SENSOR.IMU3.accel_y) || ...
    hasChanged(IN_SENSOR.IMU3.accel_z);
    updateFlag.baro1 = hasChanged(IN_SENSOR.baro1.alt_baro);
    settings: executionOrder=1
  state OUTPUT [parallel] [commented out]
    du:
    % 信号更新
    SensorIntegrityInfo.SensorUpdateFlag = updateFlag;
    % 传感器选择
    SensorIntegrityInfo.SensorSelect = SensorSelect;
    % 信号丢失信息
    SensorIntegrityInfo.sensorLostTime = sensorLostTime;
    % 信号丢失信息
    SensorIntegrityInfo.SensorStatus = SensorStatus;
  data: flag function_output; flag function_output; flag function_output; flag function_output; flag function_output; flag function_output; flag function_output; flag function_output; flag function_output; flag function_output; IN_SENSOR input Bus: BUS_SENSOR; updateFlag output Bus: BUS_NAVI_SensorSignalIntegrity_SensorUpdateFlag
  function flag = isMeasureAbnormal:
    | function flag = isMeasureAbnormal
    | flag = false;
  function flag = isMeasureAbnormal:
    | function flag = isMeasureAbnormal
    | flag = false;
  function flag = isMeasureAbnormal:
    | function flag = isMeasureAbnormal
    | flag = false;
  function flag = isMeasureAbnormal:
    | function flag = isMeasureAbnormal
    | persistent normMag_pre maxMag_pre minMag_pre
    | if isempty(normMag_pre)
    |     normMag_pre = 0.55;
    |     maxMag_pre = 0.55;
    |     minMag_pre = 0.55;
    | end
    | normMag = double(norm([IN_SENSOR.mag1.mag_x,IN_SENSOR.mag1.mag_y,IN_SENSOR.mag1.mag_z]));
    | if normMag < minMag_pre % 更新最小值
    |     minMag_pre = normMag;
    | end
    | if normMag > maxMag_pre % 更新最大值
    |     maxMag_pre = normMag;
    | end
    | flag = false;
    | if normMag < SENSOR_INTEGRITY_PARAM.Mag.threshold_minNormMag_uT || ...
    |         normMag > SENSOR_INTEGRITY_PARAM.Mag.threshold_maxNormMag_uT || ...
    |            maxMag_pre - normMag_pre > SENSOR_INTEGRITY_PARAM.Mag.threshold_gapBetweenMaxMin_uT
    |     flag = true; 
    | end
    | normMag_pre = normMag;
  function flag = isMeasureAbnormal:
    | function flag = isMeasureAbnormal
    | persistent normMag_pre maxMag_pre minMag_pre
    | if isempty(normMag_pre)
    |     normMag_pre = 0.55;
    |     maxMag_pre = 0.55;
    |     minMag_pre = 0.55;
    | end
    | normMag = double(norm([IN_SENSOR.mag2.mag_x,IN_SENSOR.mag2.mag_y,IN_SENSOR.mag2.mag_z]));
    | if normMag < minMag_pre % 更新最小值
    |     minMag_pre = normMag;
    | end
    | if normMag > maxMag_pre % 更新最大值
    |     maxMag_pre = normMag;
    | end
    | flag = false;
    | if normMag < SENSOR_INTEGRITY_PARAM.Mag.threshold_minNormMag_uT || ...
    |         normMag > SENSOR_INTEGRITY_PARAM.Mag.threshold_maxNormMag_uT || ...
    |            maxMag_pre - normMag_pre > SENSOR_INTEGRITY_PARAM.Mag.threshold_gapBetweenMaxMin_uT
    |     flag = true; 
    | end
    | normMag_pre = normMag;
  function flag = isMeasureAbnormal:
    | function flag = isMeasureAbnormal
    | persistent lat_pre lon_pre speed_pre
    | tempGPS = IN_SENSOR.ublox1;
    | curLat = double(tempGPS.Lat);
    | curLon = double(tempGPS.Lon);
    | curSpeed = double(norm([tempGPS.velN,tempGPS.velE,tempGPS.velD]));
    | if isempty(lat_pre)
    |     lat_pre = curLat;
    |     lon_pre = curLon;
    |     speed_pre = curSpeed;
    | end
    | 
    | flag = false;
    | if tempGPS.numSv < SENSOR_INTEGRITY_PARAM.GPS.threshold_numSv || ...
    |         tempGPS.pDop > SENSOR_INTEGRITY_PARAM.GPS.threshold_pDop || ...
    |         abs(lat_pre-curLat) > 5e-4 || ...
    |         abs(lon_pre-curLon) > 5e-4 || ...
    |         abs(speed_pre-curSpeed) > 20
    |     flag = true; 
    | end
    | 
    | lat_pre = curLat;
    | lon_pre = curLon;
    | speed_pre = curSpeed;
  function flag = isMeasureAbnormal:
    | function flag = isMeasureAbnormal
    | persistent lat_pre lon_pre speed_pre
    | tempGPS = IN_SENSOR.um482;
    | curLat = double(tempGPS.Lat);
    | curLon = double(tempGPS.Lon);
    | curSpeed = double(norm([tempGPS.velN,tempGPS.velE,tempGPS.velD]));
    | if isempty(lat_pre)
    |     lat_pre = curLat;
    |     lon_pre = curLon;
    |     speed_pre = curSpeed;
    | end
    | 
    | flag = false;
    | if tempGPS.numSv < SENSOR_INTEGRITY_PARAM.GPS.threshold_numSv || ...
    |         tempGPS.pDop > SENSOR_INTEGRITY_PARAM.GPS.threshold_pDop || ...
    |         abs(lat_pre-curLat) > 5e-4 || ...
    |         abs(lon_pre-curLon) > 5e-4 || ...
    |         abs(speed_pre-curSpeed) > 20
    |     flag = true; 
    | end
    | 
    | lat_pre = curLat;
    | lon_pre = curLon;
    | speed_pre = curSpeed;
  function flag = isMeasureAbnormal:
    | function flag = isMeasureAbnormal
    | flag = false;
  function flag = isMeasureAbnormal:
    | function flag = isMeasureAbnormal
    | flag = false;
  function flag = isMeasureAbnormal:
    | function flag = isMeasureAbnormal
    | flag = false;
